simulink model "sampleModel106"  (R2022a)
settings: Solver=VariableStepAuto  StartTime=0.0  StopTime=10.0  RelTol=1e-3
undefined symbols (not defined in the file): DiscIntNeverNeededParam, magnitude, Newton, Raphson
libraries: simulink x379, slpidlib x89
(part 4 of 16)

== system sampleModel106/cfblk79/cfblk7/cfblk10 ==
  cfblk1 : Inport
  cfblk10 : Constant  Value=[930798698.879540]  SampleTime=1
  cfblk11 : Constant  Value=[942896576.125749]  SampleTime=1
  cfblk12 : Subsystem
  cfblk13 : Subsystem
  cfblk14 : Subsystem
  cfblk{15..18} (4 alike) : Delay  SampleTime=1
  cfblk3 : slpidlib/PID Controller (2DOF)  Controller=PID  Form=Parallel  TimeDomain=Discrete-time  UseExternalTs=off  SampleTime=1  IntegratorMethod=Forward Euler  FilterMethod=Forward Euler  ControllerParametersSource=internal  P=1  I=1  UseKiTs=off  D=0  N=100  UseFilter=on  b=1  c=1  TunerSelectOption=Transfer Function Based (PID Tuner App)  InitialConditionSource=internal  InitialConditionForIntegrator=0  InitialConditionForFilter=0  DifferentiatorICPrevScaledInput=0  ExternalReset=none  TrackingMode=off  Kt=1  LimitOutput=off  SatLimitsSource=internal  UpperSaturationLimit=inf  LowerSaturationLimit=-inf  LinearizeAsGain=off  AntiWindupMode=none  Kb=1  POutMin=[]  POutMax=[]  IOutMin=[]  IOutMax=[]  DOutMin=[]  DOutMax=[]  NOutMin=[]  NOutMax=[]  bOutMin=[]  bOutMax=[]  cOutMin=[]  cOutMax=[]  SumOutMin=[]  SumOutMax=[]  SaturationOutMin=[]  SaturationOutMax=[]  PParamMin=[]  PParamMax=[]  IParamMin=[]  IParamMax=[]  DParamMin=[]  DParamMax=[]  NParamMin=[]  NParamMax=[]  bParamMin=[]  bParamMax=[]  cParamMin=[]  cParamMax=[]  KbParamMin=[]  KbParamMax=[]  KtParamMin=[]  KtParamMax=[]  KbOutMin=[]  KbOutMax=[]  KtOutMin=[]  KtOutMax=[]  IntegratorOutMin=[]  IntegratorOutMax=[]  FilterOutMin=[]  FilterOutMax=[]  SumI1OutMin=[]  SumI1OutMax=[]  SumI2OutMin=[]  SumI2OutMax=[]  SumI3OutMin=[]  SumI3OutMax=[]  SumI4OutMin=[]  SumI4OutMax=[]  SumDOutMin=[]  SumDOutMax=[]  Sum1OutMin=[]  Sum1OutMax=[]  Sum2OutMin=[]  Sum2OutMax=[]  Sum3OutMin=[]  Sum3OutMax=[]  DifferentiatorOutMin=[]  DifferentiatorOutMax=[]  FilterDiffOutCoefMin=[]  FilterDiffOutCoefMax=[]  ReciprocalOutMin=[]  ReciprocalOutMax=[]  SumDenOutMin=[]  SumDenOutMax=[]  SumNumOutMin=[]  SumNumOutMax=[]  DivideOutMin=[]  DivideOutMax=[]  UdiffTsProdOutMin=[]  UdiffTsProdOutMax=[]  NTsProdOutMin=[]  NTsProdOutMax=[]  UintegralTsProdOutMin=[]  UintegralTsProdOutMax=[]  UngainTsProdOutMin=[]  UngainTsProdOutMax=[]  IntegratorContinuousStateAttributes=''  IntegratorStateMustResolveToSignalObject=off  IntegratorRTWStateStorageClass=Auto  FilterContinuousStateAttributes=''  FilterStateMustResolveToSignalObject=off  FilterRTWStateStorageClass=Auto  ParallelPVariant=InternalParameters  IdealPVariant=Disabled  IVariant=InternalParameters  DVariant=InternalParameters  bVariant=InternalParameters  cVariant=InternalParameters  IntegratorVariant=Discrete  SatVariant=Disabled  AWVariant=Passthrough  PCopyVariant=Disabled  TRVariant=Disabled  FdbkBlocksVariant=Forward  IdealPFdbkVariant=Disabled  SatFdbkVariant=Disabled  DerivativeFilterVariant=ForwardEulerFilter  NVariant=InternalParameters  NCopyVariant=Disabled  FilterICVariant=InternalICsFilter  IntegratorICVariant=InternalICs  ExternalResetVariant=Disabled  TRSumVariant=Passthrough  SumFdbkVariant=Disabled  SumVariant=Sum_PID  TsampFilterVariant=InternalTs  TsampNgainVariant=Passthrough  TsampIntegralVariant=Passthrough  ExternalSaturationOutDataTypeStr=Inherit: Same as second input
      settings: SourceProductBaseCode=SL
  cfblk4 : simulink/Discrete/Transfer Fcn Real Zero  ZeroZ=0.75  ICPrevInput=0.0  DoSatur=off
      settings: SourceProductBaseCode=SL
  cfblk5 : simulink/Discrete/Transfer Fcn First Order  PoleZ=0.95  ICPrevOutput=0.0  DoSatur=off
  cfblk6 : Sqrt
  cfblk7 : Sqrt
  cfblk8 : simulink/Math Operations/Slider Gain  gain=1  low=0  high=2
  cfblk9 : Bias  Bias=[-914547020.820806]  SaturateOnIntegerOverflow=off
  cfblk2 : Outport
  wires:
  cfblk5/1 -> cfblk9/1, cfblk12/2(cfblk9)
  cfblk7/1 -> cfblk4/1
  cfblk12/1(cfblk2) -> cfblk13/1(cfblk1)
  cfblk1/1 -> cfblk14/1(cfblk1)
  cfblk14/1(cfblk2) -> cfblk7/1
  cfblk13/1(cfblk2) -> cfblk3/1
  cfblk8/1 -> cfblk13/2(cfblk16)
  cfblk10/1 -> cfblk8/1
  cfblk9/1 -> cfblk6/1, cfblk18/1
  cfblk11/1 -> cfblk13/3(cfblk17)
  cfblk14/2(cfblk16) -> cfblk5/1
  cfblk14/3(cfblk17) -> cfblk3/2
  cfblk12/2(cfblk11) -> cfblk2/1
  cfblk4/1 -> cfblk12/1(cfblk1), cfblk12/3(cfblk10)
  cfblk3/1 -> cfblk15/1
  cfblk15/1 -> cfblk14/2(cfblk12)
  cfblk12/3(cfblk12) -> cfblk16/1
  cfblk16/1 -> cfblk14/4(cfblk14)
  cfblk6/1 -> cfblk17/1
  cfblk17/1 -> cfblk14/3(cfblk13)
  cfblk18/1 -> cfblk14/5(cfblk15)

== system sampleModel106/cfblk79/cfblk7/cfblk11 ==
  cfblk1 : Inport
  cfblk13 : Inport  Port=2
  cfblk14 : Inport  Port=3
  cfblk10 : Subsystem
  cfblk11 : Subsystem
  cfblk12 : Subsystem
  cfblk18 : Delay  SampleTime=1
  cfblk3 : simulink/Discrete/Transfer Fcn First Order  PoleZ=0.95  ICPrevOutput=0.0  DoSatur=off
  cfblk4 : Sqrt
  cfblk5 : Constant  Value=[-218946941.041430]  SampleTime=1
  cfblk6 : Constant  Value=[703044914.610683]  SampleTime=1
  cfblk7 : Constant  Value=[340158216.869012]  SampleTime=1
  cfblk8 : Constant  Value=[55648413.249553]  SampleTime=1
  cfblk9 : Subsystem
  cfblk2 : Outport
  cfblk15 : Outport  Port=2
  cfblk16 : Outport  Port=3
  cfblk17 : Outport  Port=4
  wires:
  cfblk9/1(cfblk2) -> cfblk12/1(cfblk1)
  cfblk1/1 -> cfblk3/1
  cfblk7/1 -> cfblk16/1
  cfblk9/2(cfblk13) -> cfblk11/1(cfblk1)
  cfblk9/3(cfblk14) -> cfblk4/1
  cfblk5/1 -> cfblk17/1, cfblk9/3(cfblk12)
  cfblk14/1 -> cfblk11/2(cfblk11)
  cfblk11/1(cfblk2) -> cfblk15/1
  cfblk11/2(cfblk13) -> cfblk10/1(cfblk1)
  cfblk6/1 -> cfblk2/1
  cfblk4/1 -> cfblk11/3(cfblk12), cfblk12/3(cfblk14)
  cfblk13/1 -> cfblk10/2(cfblk12)
  cfblk12/1(cfblk2) -> cfblk10/3(cfblk13)
  cfblk3/1 -> cfblk9/1(cfblk1)
  cfblk8/1 -> cfblk9/2(cfblk11)
  cfblk10/1(cfblk2) -> cfblk18/1
  cfblk18/1 -> cfblk12/2(cfblk13)

== system sampleModel106/cfblk79/cfblk7/cfblk12 ==
  cfblk1 : Inport
  cfblk15 : Inport  Port=2
  cfblk16 : Inport  Port=3
  cfblk10 : Constant  Value=[896827998.321361]  SampleTime=1
  cfblk11 : Subsystem
  cfblk12 : Subsystem
  cfblk13 : Subsystem
  cfblk14 : Subsystem
  cfblk{18..22} (5 alike) : Delay  SampleTime=1
  cfblk3 : ComplexToMagnitudeAngle
  cfblk4 : Product
  cfblk5 : Gain  Gain=[-931939284.867982]
  cfblk6 : simulink/Math Operations/MinMax Running Resettable  Function=min  vinit=0.0
  cfblk7 : Bias  Bias=[-319907071.485030]  SaturateOnIntegerOverflow=off
  cfblk8 : Sum  Inputs=+-
  cfblk9 : Constant  Value=[-736006589.998858]  SampleTime=1
  cfblk2 : Outport
  cfblk17 : Outport  Port=2
  wires:
  cfblk6/1 -> cfblk11/1(cfblk1)
  cfblk15/1 -> cfblk11/2(cfblk9)
  cfblk5/1 -> cfblk2/1
  cfblk1/1 -> cfblk3/1
  cfblk16/1 -> cfblk5/1
  cfblk3/1 -> cfblk17/1
  cfblk9/1 -> cfblk14/1(cfblk1)
  cfblk14/1(cfblk2) -> cfblk13/1(cfblk1)
  cfblk8/1 -> cfblk4/1
  cfblk3/2 -> cfblk8/2
  cfblk14/2(cfblk14) -> cfblk12/1(cfblk1)
  cfblk13/2(cfblk11) -> cfblk4/2
  cfblk13/3(cfblk12) -> cfblk7/1
  cfblk11/1(cfblk2) -> cfblk14/2(cfblk12)
  cfblk4/1 -> cfblk18/1
  cfblk18/1 -> cfblk8/1
  cfblk13/1(cfblk2) -> cfblk19/1
  cfblk19/1 -> cfblk6/1
  cfblk7/1 -> cfblk20/1
  cfblk20/1 -> cfblk13/2(cfblk10)
  cfblk12/1(cfblk2) -> cfblk21/1
  cfblk21/1 -> cfblk14/3(cfblk13)
  cfblk14/3(cfblk15) -> cfblk22/1
  cfblk22/1 -> cfblk6/2

== system sampleModel106/cfblk79/cfblk7/cfblk13 ==
  cfblk1 : Inport
  cfblk10 : Subsystem  TreatAsAtomicUnit=on
  cfblk{11..14} (4 alike) : Delay  SampleTime=1
  cfblk3 : MinMax  Inputs=2
  cfblk4 : PermuteDimensions
  cfblk5 : Constant  Value=[199750980.008427]  SampleTime=1
  cfblk6 : Subsystem
  cfblk7 : Subsystem
  cfblk8 : If  IfExpression=u1 >= 0  SampleTime=1
  cfblk9 : Subsystem  TreatAsAtomicUnit=on
  cfblk2 : Outport
  wires:
  cfblk3/1 -> cfblk10/1(cfblk1)
  cfblk10/1(cfblk2) -> cfblk2/1
  cfblk4/1 -> cfblk9/2(cfblk13)
  cfblk5/1 -> cfblk6/1(cfblk1)
  cfblk1/1 -> cfblk10/2(cfblk8)
  cfblk9/2(cfblk14) -> cfblk7/1(cfblk1)
  cfblk9/3(cfblk15) -> cfblk7/2(cfblk11)
  cfblk7/2(cfblk12) -> cfblk3/1
  cfblk6/2(cfblk7) -> cfblk3/2
  cfblk7/3(cfblk13) -> cfblk6/2(cfblk6)
  cfblk8/1 -> cfblk9/Action
  cfblk8/2 -> cfblk10/Action
  cfblk9/1(cfblk2) -> cfblk11/1
  cfblk11/1 -> cfblk4/1
  cfblk7/1(cfblk2) -> cfblk12/1
  cfblk12/1 -> cfblk9/1(cfblk1)
  cfblk6/1(cfblk2) -> cfblk13/1
  cfblk13/1 -> cfblk8/1
  cfblk7/4(cfblk14) -> cfblk14/1
  cfblk14/1 -> cfblk10/3(cfblk9)

== system sampleModel106/cfblk79/cfblk8/cfblk10 ==
  cfblk1 : Inport
  cfblk{3,11..17} (8 alike) : Delay  SampleTime=1
  cfblk4 : Delay  ShowEnablePort=on  SampleTime=1
      settings: InputPortMap=u0,e6
  cfblk5 : Abs  SaturateOnIntegerOverflow=off
  cfblk6 : Sqrt  Operator=rSqrt  AlgorithmType=Newton-Raphson
  cfblk7 : Subsystem
  cfblk8 : Subsystem
  cfblk2 : Outport
  cfblk9 : Outport  Port=2
  cfblk10 : Outport  Port=3
  wires:
  cfblk3/1 -> cfblk9/1
  cfblk6/1 -> cfblk5/1, cfblk2/1, cfblk16/1, cfblk17/1
  cfblk5/1 -> cfblk4/1, cfblk4/2, cfblk11/1, cfblk12/1
  cfblk1/1 -> cfblk7/2(cfblk6), cfblk8/3(cfblk10)
  cfblk7/1(cfblk2) -> cfblk8/1(cfblk1)
  cfblk8/1(cfblk2) -> cfblk10/1
  cfblk8/2(cfblk13) -> cfblk6/1
  cfblk8/3(cfblk14) -> cfblk3/1
  cfblk4/1 -> cfblk13/1, cfblk14/1, cfblk15/1
  cfblk11/1 -> cfblk7/1(cfblk1)
  cfblk12/1 -> cfblk7/3(cfblk7)
  cfblk13/1 -> cfblk8/2(cfblk9)
  cfblk14/1 -> cfblk8/4(cfblk11)
  cfblk15/1 -> cfblk7/5(cfblk9)
  cfblk16/1 -> cfblk8/5(cfblk12)
  cfblk17/1 -> cfblk7/4(cfblk8)

== system sampleModel106/cfblk79/cfblk8/cfblk11 ==
  cfblk1 : Inport
  cfblk14 : Inport  Port=2
  cfblk10 : Constant  Value=[476735084.227902]  SampleTime=1
  cfblk11 : Subsystem
  cfblk12 : Subsystem
  cfblk13 : If  IfExpression=u1 >= 0  SampleTime=1
  cfblk18 : Subsystem  TreatAsAtomicUnit=on
  cfblk19 : Subsystem  TreatAsAtomicUnit=on
  cfblk20 : Delay  SampleTime=1
  cfblk21 : Delay  SampleTime=1
  cfblk22 : Delay  SampleTime=1
  cfblk3 : simulink/Discrete/Transfer Fcn Real Zero  ZeroZ=0.75  ICPrevInput=0.0  DoSatur=off
      settings: SourceProductBaseCode=SL
  cfblk4 : Product  Inputs=**
  cfblk5 : Sqrt  Operator=rSqrt  AlgorithmType=Newton-Raphson
  cfblk6 : Signum
  cfblk7 : Signum
  cfblk8 : Sum  Inputs=+
  cfblk9 : Constant  Value=[-437500950.255498]  SampleTime=1
  cfblk2 : Outport
  cfblk15 : Outport  Port=2
  cfblk16 : Outport  Port=3
  cfblk17 : Outport  Port=4
  wires:
  cfblk8/1 -> cfblk11/1(cfblk1)
  cfblk3/1 -> cfblk5/1, cfblk11/3(cfblk13)
  cfblk7/1 -> cfblk15/1, cfblk21/1
  cfblk19/1(cfblk2) -> cfblk4/1
  cfblk19/2(cfblk13) -> cfblk16/1
  cfblk6/1 -> cfblk13/1
  cfblk12/1(cfblk2) -> cfblk7/1
  cfblk12/2(cfblk10) -> cfblk2/1
  cfblk19/3(cfblk14) -> cfblk17/1
  cfblk11/1(cfblk2) -> cfblk4/2
  cfblk10/1 -> cfblk8/1, cfblk19/3(cfblk12)
  cfblk19/4(cfblk15) -> cfblk3/1, cfblk11/4(cfblk14)
  cfblk5/1 -> cfblk12/1(cfblk1), cfblk11/6(cfblk16)
  cfblk18/1(cfblk2) -> cfblk11/2(cfblk12)
  cfblk14/1 -> cfblk12/2(cfblk9)
  cfblk1/1 -> cfblk6/1, cfblk11/5(cfblk15)
  cfblk9/1 -> cfblk19/2(cfblk11)
  cfblk13/1 -> cfblk18/Action
  cfblk13/2 -> cfblk19/Action
  cfblk4/1 -> cfblk20/1
  cfblk20/1 -> cfblk18/2(cfblk8)
  cfblk21/1 -> cfblk18/1(cfblk1)
  cfblk12/3(cfblk11) -> cfblk22/1
  cfblk22/1 -> cfblk19/1(cfblk1)

== system sampleModel106/cfblk79/cfblk8/cfblk9 ==
  cfblk1 : Inport
  cfblk10 : Inport  Port=2
  cfblk11 : Inport  Port=3
  cfblk12 : Inport  Port=4
  cfblk13 : Delay  SampleTime=1
  cfblk14 : Delay  SampleTime=1
  cfblk3 : simulink/Math Operations/MinMax Running Resettable  Function=min  vinit=0.0
  cfblk4 : Sqrt  Operator=rSqrt  AlgorithmType=Newton-Raphson
  cfblk5 : Signum
  cfblk6 : Polyval  Coefs=[ +2.081618890e-019, -1.441693666e-014, +4.719686976e-010, -8.536869453e-006, +1.621573104e-001, -8.087801117e+001 ]
  cfblk7 : Abs  SaturateOnIntegerOverflow=off
  cfblk8 : Sum  Inputs=--
  cfblk9 : Subsystem
  cfblk2 : Outport
  wires:
  cfblk11/1 -> cfblk2/1
  cfblk10/1 -> cfblk3/1
  cfblk4/1 -> cfblk6/1
  cfblk12/1 -> cfblk9/1(cfblk1)
  cfblk9/1(cfblk2) -> cfblk4/1
  cfblk8/1 -> cfblk3/2
  cfblk7/1 -> cfblk8/1
  cfblk6/1 -> cfblk8/2, cfblk14/1
  cfblk9/2(cfblk10) -> cfblk7/1
  cfblk1/1 -> cfblk5/1
  cfblk5/1 -> cfblk9/2(cfblk7)
  cfblk3/1 -> cfblk13/1
  cfblk13/1 -> cfblk9/3(cfblk8)
  cfblk14/1 -> cfblk9/4(cfblk9)

== system sampleModel106/cfblk80/cfblk10/cfblk10 ==
  cfblk1 : Inport
  cfblk13 : Inport  Port=2
  cfblk10 : Subsystem
  cfblk11 : Subsystem
  cfblk12 : Subsystem
  cfblk15 : Delay  SampleTime=1
  cfblk16 : Delay  SampleTime=1
  cfblk17 : Delay  SampleTime=1
  cfblk3 : ComplexToRealImag
  cfblk4 : Product  Inputs=*
  cfblk5 : simulink/Math Operations/Slider Gain  gain=1  low=0  high=2
  cfblk6 : PermuteDimensions
  cfblk7 : Trigonometry
  cfblk8 : Constant  Value=[898456945.035176]  SampleTime=1
  cfblk9 : Subsystem
  cfblk2 : Outport
  cfblk14 : Outport  Port=2
  wires:
  cfblk1/1 -> cfblk9/1(cfblk1)
  cfblk13/1 -> cfblk5/1
  cfblk10/1(cfblk2) -> cfblk12/1(cfblk1)
  cfblk10/2(cfblk7) -> cfblk7/1
  cfblk12/1(cfblk2) -> cfblk4/1
  cfblk8/1 -> cfblk11/1(cfblk1)
  cfblk9/1(cfblk2) -> cfblk6/1
  cfblk11/1(cfblk2) -> cfblk12/2(cfblk6), cfblk14/1
  cfblk6/1 -> cfblk10/1(cfblk1)
  cfblk5/1 -> cfblk2/1, cfblk3/1
  cfblk3/1 -> cfblk12/3(cfblk7)
  cfblk3/2 -> cfblk12/4(cfblk8), cfblk11/2(cfblk9)
  cfblk4/1 -> cfblk15/1
  cfblk15/1 -> cfblk9/3(cfblk13)
  cfblk12/2(cfblk9) -> cfblk16/1
  cfblk16/1 -> cfblk10/2(cfblk6)
  cfblk7/1 -> cfblk17/1
  cfblk17/1 -> cfblk9/2(cfblk12)

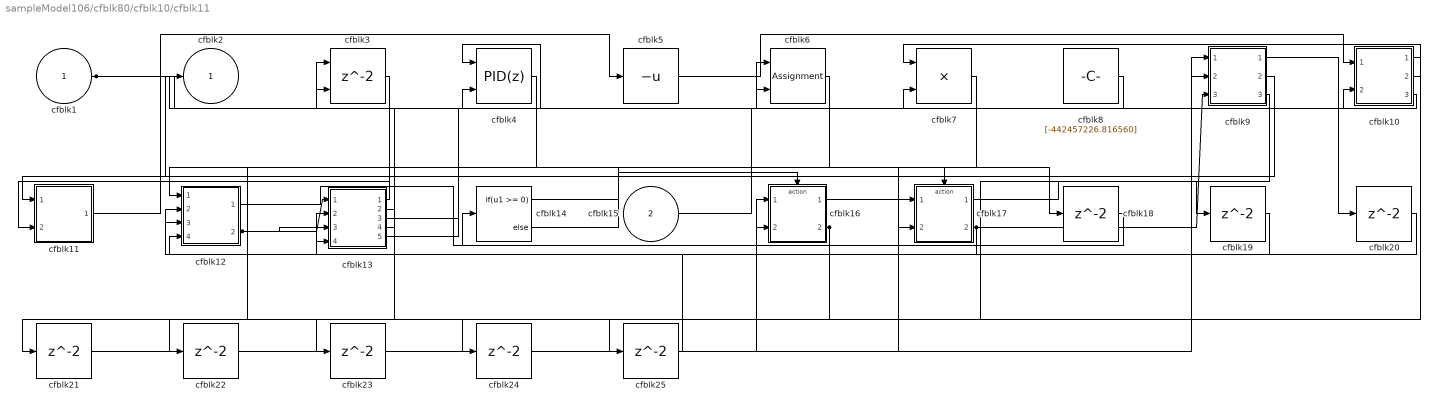
== system sampleModel106/cfblk80/cfblk10/cfblk11 ==
  cfblk1 : Inport
  cfblk15 : Inport  Port=2
  cfblk10 : Subsystem
  cfblk11 : Subsystem
  cfblk12 : Subsystem
  cfblk13 : Subsystem
  cfblk14 : If  IfExpression=u1 >= 0  SampleTime=1
  cfblk16 : Subsystem  TreatAsAtomicUnit=on
  cfblk17 : Subsystem  TreatAsAtomicUnit=on
  cfblk{18..25} (8 alike) : Delay  SampleTime=1
  cfblk3 : Delay  ShowEnablePort=on  SampleTime=1
      settings: InputPortMap=u0,e6
  cfblk4 : slpidlib/PID Controller (2DOF)  Controller=PID  Form=Parallel  TimeDomain=Discrete-time  UseExternalTs=off  SampleTime=1  IntegratorMethod=Forward Euler  FilterMethod=Forward Euler  ControllerParametersSource=internal  P=1  I=1  UseKiTs=off  D=0  N=100  UseFilter=on  b=1  c=1  TunerSelectOption=Transfer Function Based (PID Tuner App)  InitialConditionSource=internal  InitialConditionForIntegrator=0  InitialConditionForFilter=0  DifferentiatorICPrevScaledInput=0  ExternalReset=none  TrackingMode=off  Kt=1  LimitOutput=off  SatLimitsSource=internal  UpperSaturationLimit=inf  LowerSaturationLimit=-inf  LinearizeAsGain=off  AntiWindupMode=none  Kb=1  POutMin=[]  POutMax=[]  IOutMin=[]  IOutMax=[]  DOutMin=[]  DOutMax=[]  NOutMin=[]  NOutMax=[]  bOutMin=[]  bOutMax=[]  cOutMin=[]  cOutMax=[]  SumOutMin=[]  SumOutMax=[]  SaturationOutMin=[]  SaturationOutMax=[]  PParamMin=[]  PParamMax=[]  IParamMin=[]  IParamMax=[]  DParamMin=[]  DParamMax=[]  NParamMin=[]  NParamMax=[]  bParamMin=[]  bParamMax=[]  cParamMin=[]  cParamMax=[]  KbParamMin=[]  KbParamMax=[]  KtParamMin=[]  KtParamMax=[]  KbOutMin=[]  KbOutMax=[]  KtOutMin=[]  KtOutMax=[]  IntegratorOutMin=[]  IntegratorOutMax=[]  FilterOutMin=[]  FilterOutMax=[]  SumI1OutMin=[]  SumI1OutMax=[]  SumI2OutMin=[]  SumI2OutMax=[]  SumI3OutMin=[]  SumI3OutMax=[]  SumI4OutMin=[]  SumI4OutMax=[]  SumDOutMin=[]  SumDOutMax=[]  Sum1OutMin=[]  Sum1OutMax=[]  Sum2OutMin=[]  Sum2OutMax=[]  Sum3OutMin=[]  Sum3OutMax=[]  DifferentiatorOutMin=[]  DifferentiatorOutMax=[]  FilterDiffOutCoefMin=[]  FilterDiffOutCoefMax=[]  ReciprocalOutMin=[]  ReciprocalOutMax=[]  SumDenOutMin=[]  SumDenOutMax=[]  SumNumOutMin=[]  SumNumOutMax=[]  DivideOutMin=[]  DivideOutMax=[]  UdiffTsProdOutMin=[]  UdiffTsProdOutMax=[]  NTsProdOutMin=[]  NTsProdOutMax=[]  UintegralTsProdOutMin=[]  UintegralTsProdOutMax=[]  UngainTsProdOutMin=[]  UngainTsProdOutMax=[]  IntegratorContinuousStateAttributes=''  IntegratorStateMustResolveToSignalObject=off  IntegratorRTWStateStorageClass=Auto  FilterContinuousStateAttributes=''  FilterStateMustResolveToSignalObject=off  FilterRTWStateStorageClass=Auto  ParallelPVariant=InternalParameters  IdealPVariant=Disabled  IVariant=InternalParameters  DVariant=InternalParameters  bVariant=InternalParameters  cVariant=InternalParameters  IntegratorVariant=Discrete  SatVariant=Disabled  AWVariant=Passthrough  PCopyVariant=Disabled  TRVariant=Disabled  FdbkBlocksVariant=Forward  IdealPFdbkVariant=Disabled  SatFdbkVariant=Disabled  DerivativeFilterVariant=ForwardEulerFilter  NVariant=InternalParameters  NCopyVariant=Disabled  FilterICVariant=InternalICsFilter  IntegratorICVariant=InternalICs  ExternalResetVariant=Disabled  TRSumVariant=Passthrough  SumFdbkVariant=Disabled  SumVariant=Sum_PID  TsampFilterVariant=InternalTs  TsampNgainVariant=Passthrough  TsampIntegralVariant=Passthrough  ExternalSaturationOutDataTypeStr=Inherit: Same as second input
      settings: SourceProductBaseCode=SL
  cfblk5 : UnaryMinus
  cfblk6 : Assignment  DiagnosticForDimensions=Warning  IndexOptions=Index vector (dialog)  Indices=1  OutputSizes=1
  cfblk7 : Product  Inputs=**
  cfblk8 : Constant  Value=[-442457226.816560]  SampleTime=1
  cfblk9 : Subsystem
  cfblk2 : Outport
  wires:
  cfblk4/1 -> cfblk12/1(cfblk1)
  cfblk8/1 -> cfblk4/1
  cfblk11/1(cfblk2) -> cfblk5/1
  cfblk16/2(cfblk14) -> cfblk13/2(cfblk6), cfblk25/1
  cfblk5/1 -> cfblk10/1(cfblk1)
  cfblk1/1 -> cfblk4/2, cfblk17/2(cfblk11)
  cfblk12/1(cfblk2) -> cfblk16/1(cfblk1)
  cfblk10/2(cfblk11) -> cfblk7/1
  cfblk13/1(cfblk2) -> cfblk2/1
  cfblk9/2(cfblk9) -> cfblk11/1(cfblk1)
  cfblk15/1 -> cfblk10/2(cfblk10)
  cfblk17/2(cfblk12) -> cfblk9/3(cfblk8), cfblk13/4(cfblk8)
  cfblk13/2(cfblk9) -> cfblk3/1
  cfblk10/3(cfblk12) -> cfblk6/1
  cfblk13/3(cfblk10) -> cfblk6/2
  cfblk13/4(cfblk11) -> cfblk3/2
  cfblk13/5(cfblk12) -> cfblk7/2
  cfblk12/2(cfblk13) -> cfblk13/1(cfblk1), cfblk13/3(cfblk7)
  cfblk3/1 -> cfblk11/2(cfblk9)
  cfblk14/1 -> cfblk16/Action
  cfblk14/2 -> cfblk17/Action
  cfblk16/1(cfblk2) -> cfblk18/1
  cfblk18/1 -> cfblk14/1
  cfblk17/1(cfblk2) -> cfblk19/1
  cfblk19/1 -> cfblk12/3(cfblk11)
  cfblk9/1(cfblk2) -> cfblk20/1
  cfblk20/1 -> cfblk12/4(cfblk12)
  cfblk10/1(cfblk2) -> cfblk21/1
  cfblk21/1 -> cfblk9/2(cfblk7)
  cfblk7/1 -> cfblk22/1
  cfblk22/1 -> cfblk9/1(cfblk1)
  cfblk6/1 -> cfblk23/1
  cfblk23/1 -> cfblk16/2(cfblk13)
  cfblk9/3(cfblk10) -> cfblk24/1
  cfblk24/1 -> cfblk17/1(cfblk1)
  cfblk25/1 -> cfblk12/2(cfblk10)

== system sampleModel106/cfblk80/cfblk10/cfblk12 ==
  cfblk1 : Inport
  cfblk3 : Delay  ShowEnablePort=on  SampleTime=1
      settings: InputPortMap=u0,e6
  cfblk4 : Delay  ShowEnablePort=on  SampleTime=1
      settings: InputPortMap=u0,e6
  cfblk5 : slpidlib/PID Controller  Controller=PID  Form=Parallel  TimeDomain=Discrete-time  UseExternalTs=off  SampleTime=1  IntegratorMethod=Forward Euler  FilterMethod=Forward Euler  ControllerParametersSource=internal  P=1  I=1  UseKiTs=off  D=0  N=100  UseFilter=on  TunerSelectOption=Transfer Function Based (PID Tuner App)  InitialConditionSource=internal  InitialConditionForIntegrator=0  InitialConditionForFilter=0  DifferentiatorICPrevScaledInput=0  ExternalReset=none  TrackingMode=off  Kt=1  LimitOutput=off  SatLimitsSource=internal  UpperSaturationLimit=inf  LowerSaturationLimit=-inf  LinearizeAsGain=off  AntiWindupMode=none  Kb=1  POutMin=[]  POutMax=[]  IOutMin=[]  IOutMax=[]  DOutMin=[]  DOutMax=[]  NOutMin=[]  NOutMax=[]  SumOutMin=[]  SumOutMax=[]  SaturationOutMin=[]  SaturationOutMax=[]  PParamMin=[]  PParamMax=[]  IParamMin=[]  IParamMax=[]  DParamMin=[]  DParamMax=[]  NParamMin=[]  NParamMax=[]  KbParamMin=[]  KbParamMax=[]  KtParamMin=[]  KtParamMax=[]  KbOutMin=[]  KbOutMax=[]  KtOutMin=[]  KtOutMax=[]  IntegratorOutMin=[]  IntegratorOutMax=[]  FilterOutMin=[]  FilterOutMax=[]  SumI1OutMin=[]  SumI1OutMax=[]  SumI2OutMin=[]  SumI2OutMax=[]  SumI3OutMin=[]  SumI3OutMax=[]  SumI4OutMin=[]  SumI4OutMax=[]  SumDOutMin=[]  SumDOutMax=[]  DifferentiatorOutMin=[]  DifferentiatorOutMax=[]  FilterDiffOutCoefMin=[]  FilterDiffOutCoefMax=[]  ReciprocalOutMin=[]  ReciprocalOutMax=[]  SumDenOutMin=[]  SumDenOutMax=[]  SumNumOutMin=[]  SumNumOutMax=[]  DivideOutMin=[]  DivideOutMax=[]  UdiffTsProdOutMin=[]  UdiffTsProdOutMax=[]  NTsProdOutMin=[]  NTsProdOutMax=[]  UintegralTsProdOutMin=[]  UintegralTsProdOutMax=[]  UngainTsProdOutMin=[]  UngainTsProdOutMax=[]  IntegratorContinuousStateAttributes=''  IntegratorStateMustResolveToSignalObject=off  IntegratorRTWStateStorageClass=Auto  FilterContinuousStateAttributes=''  FilterStateMustResolveToSignalObject=off  FilterRTWStateStorageClass=Auto  ParallelPVariant=InternalParameters  IdealPVariant=Disabled  IVariant=InternalParameters  DVariant=InternalParameters  IntegratorVariant=Discrete  SatVariant=Disabled  AWVariant=Passthrough  PCopyVariant=Disabled  TRVariant=Disabled  FdbkBlocksVariant=Forward  IdealPFdbkVariant=Disabled  SatFdbkVariant=Disabled  DerivativeFilterVariant=ForwardEulerFilter  NVariant=InternalParameters  NCopyVariant=Disabled  FilterICVariant=InternalICsFilter  IntegratorICVariant=InternalICs  ExternalResetVariant=Disabled  TRSumVariant=Passthrough  SumFdbkVariant=Disabled  SumVariant=Sum_PID  TsampFilterVariant=InternalTs  TsampNgainVariant=Passthrough  TsampIntegralVariant=Passthrough  ExternalSaturationOutDataTypeStr=Inherit: Same as second input  aMode=0
  cfblk6 : Assignment  DiagnosticForDimensions=Warning  IndexOptions=Index vector (dialog)  Indices=1  OutputSizes=1
  cfblk7 : Sum  Inputs=+-
  cfblk8 : Constant  Value=[-633710361.624369]  SampleTime=1
  cfblk9 : Subsystem
  cfblk2 : Outport
  cfblk10 : Outport  Port=2
  cfblk11 : Outport  Port=3
  wires:
  cfblk7/1 -> cfblk2/1
  cfblk9/1(cfblk2) -> cfblk3/1
  cfblk5/1 -> cfblk10/1
  cfblk4/1 -> cfblk3/2
  cfblk3/1 -> cfblk5/1
  cfblk1/1 -> cfblk7/1, cfblk6/2
  cfblk8/1 -> cfblk9/1(cfblk1), cfblk4/1, cfblk11/1
  cfblk9/2(cfblk11) -> cfblk6/1, cfblk4/2
  cfblk6/1 -> cfblk7/2

== system sampleModel106/cfblk80/cfblk10/cfblk16 ==
  cfblk1 : Inport
  cfblk7 : Inport  Port=2
  Action Port : ActionPort  ActionPortLabel=if(u1 >= 0)
  cfblk3 : PermuteDimensions
  cfblk4 : Polyval  Coefs=[ +2.081618890e-019, -1.441693666e-014, +4.719686976e-010, -8.536869453e-006, +1.621573104e-001, -8.087801117e+001 ]
  cfblk5 : Sum  Inputs=+-
  cfblk6 : Subsystem
  cfblk8 : Delay
  cfblk9 : Delay
  cfblk2 : Outport
  wires:
  cfblk4/1 -> cfblk5/1
  cfblk6/1(cfblk2) -> cfblk3/1
  cfblk1/1 -> cfblk6/1(cfblk1)
  cfblk6/2(cfblk11) -> cfblk4/1
  cfblk5/1 -> cfblk8/1, cfblk9/1
  cfblk3/1 -> cfblk2/1, cfblk5/2
  cfblk7/1 -> cfblk6/3(cfblk8), cfblk6/5(cfblk10)
  cfblk8/1 -> cfblk6/2(cfblk7)
  cfblk9/1 -> cfblk6/4(cfblk9)

== system sampleModel106/cfblk80/cfblk10/cfblk17 ==
  cfblk1 : Inport
  cfblk16 : Inport  Port=2
  Action Port : ActionPort  ActionPortLabel=else
  cfblk10 : Trigonometry
  cfblk11 : Product  Inputs=**
  cfblk12 : Constant  Value=[9296872.569103]  SampleTime=1
  cfblk13 : Subsystem
  cfblk14 : Subsystem
  cfblk15 : Subsystem
  cfblk18 : Delay
  cfblk19 : Delay
  cfblk20 : Delay
  cfblk3 : simulink/Discrete/Transfer Fcn Lead or Lag  PoleZ=0.95  ZeroZ=0.75  ICPrevOutput=0.0  ICPrevInput=0.0  DoSatur=off
      settings: SourceProductBaseCode=SL
  cfblk4 : simulink/Discrete/Transfer Fcn Lead or Lag  PoleZ=0.95  ZeroZ=0.75  ICPrevOutput=0.0  ICPrevInput=0.0  DoSatur=off
      settings: SourceProductBaseCode=SL
  cfblk5 : DiscreteZeroPole  Poles=[0 0.5]  Gain=1  SampleTime=-1
  cfblk6 : DiscreteTransferFcn
  cfblk7 : PermuteDimensions
  cfblk8 : Reshape
  cfblk9 : Sqrt  Operator=rSqrt  AlgorithmType=Newton-Raphson
  cfblk2 : Outport
  cfblk17 : Outport  Port=2
  wires:
  cfblk6/1 -> cfblk7/1, cfblk20/1
  cfblk16/1 -> cfblk13/1(cfblk1)
  cfblk13/1(cfblk2) -> cfblk10/1
  cfblk13/2(cfblk15) -> cfblk2/1, cfblk15/3(cfblk10), cfblk14/5(cfblk11)
  cfblk14/1(cfblk2) -> cfblk3/1
  cfblk7/1 -> cfblk4/1, cfblk19/1
  cfblk10/1 -> cfblk5/1
  cfblk12/1 -> cfblk14/1(cfblk1)
  cfblk11/1 -> cfblk13/2(cfblk14)
  cfblk1/1 -> cfblk11/1
  cfblk3/1 -> cfblk17/1
  cfblk5/1 -> cfblk14/2(cfblk8)
  cfblk15/1(cfblk2) -> cfblk6/1
  cfblk9/1 -> cfblk14/3(cfblk9), cfblk14/6(cfblk12)
  cfblk4/1 -> cfblk9/1, cfblk8/1
  cfblk8/1 -> cfblk14/4(cfblk10)
  cfblk14/2(cfblk13) -> cfblk18/1
  cfblk18/1 -> cfblk11/2
  cfblk19/1 -> cfblk15/2(cfblk9)
  cfblk20/1 -> cfblk15/1(cfblk1)

== system sampleModel106/cfblk80/cfblk10/cfblk7 ==
  cfblk1 : Inport
  cfblk10 : If  IfExpression=u1 >= 0  SampleTime=1
  cfblk11 : Subsystem  TreatAsAtomicUnit=on
  cfblk12 : Subsystem  TreatAsAtomicUnit=on
  cfblk{13..16} (4 alike) : Delay  SampleTime=1
  cfblk3 : simulink/Discrete/Tapped Delay  vinit=0.0  samptime=-1  NumDelays=1  DelayOrder=Oldest  includeCurrent=off
  cfblk4 : simulink/Math Operations/Slider Gain  gain=1  low=0  high=2
  cfblk5 : Sqrt
  cfblk6 : Product  Inputs=**
  cfblk7 : Subsystem
  cfblk8 : Subsystem
  cfblk9 : Subsystem
  cfblk2 : Outport
  wires:
  cfblk4/1 -> cfblk9/1(cfblk1)
  cfblk3/1 -> cfblk10/1
  cfblk7/1(cfblk2) -> cfblk8/1(cfblk1)
  cfblk11/2(cfblk12) -> cfblk12/1(cfblk1)
  cfblk1/1 -> cfblk7/1(cfblk1)
  cfblk12/1(cfblk2) -> cfblk5/1
  cfblk12/2(cfblk7) -> cfblk2/1
  cfblk9/2(cfblk12) -> cfblk6/1
  cfblk9/3(cfblk13) -> cfblk6/2
  cfblk7/2(cfblk12) -> cfblk8/2(cfblk10)
  cfblk6/1 -> cfblk8/3(cfblk11)
  cfblk10/1 -> cfblk11/Action
  cfblk10/2 -> cfblk12/Action
  cfblk8/1(cfblk2) -> cfblk13/1
  cfblk13/1 -> cfblk7/2(cfblk11)
  cfblk11/1(cfblk2) -> cfblk14/1
  cfblk14/1 -> cfblk3/1
  cfblk5/1 -> cfblk15/1
  cfblk15/1 -> cfblk11/1(cfblk1)
  cfblk9/1(cfblk2) -> cfblk16/1
  cfblk16/1 -> cfblk4/1

== system sampleModel106/cfblk80/cfblk10/cfblk8 ==
  cfblk1 : Inport
  cfblk10 : Subsystem
  cfblk11 : If  IfExpression=u1 >= 0  SampleTime=1
  cfblk12 : Subsystem  TreatAsAtomicUnit=on
  cfblk13 : Subsystem  TreatAsAtomicUnit=on
  cfblk{14..21} (8 alike) : Delay  SampleTime=1
  cfblk3 : simulink/Discrete/Transfer Fcn Real Zero  ZeroZ=0.75  ICPrevInput=0.0  DoSatur=off
      settings: SourceProductBaseCode=SL
  cfblk4 : Assignment  DiagnosticForDimensions=Warning  IndexOptions=Index vector (dialog)  Indices=1  OutputSizes=1
  cfblk5 : Constant  Value=[-476104574.584805]  SampleTime=1
  cfblk6 : Subsystem
  cfblk7 : Subsystem
  cfblk8 : Subsystem
  cfblk9 : Subsystem
  cfblk2 : Outport
  wires:
  cfblk4/1 -> cfblk8/4(cfblk9), cfblk20/1, cfblk21/1
  cfblk6/1(cfblk2) -> cfblk8/1(cfblk1)
  cfblk13/1(cfblk2) -> cfblk2/1
  cfblk1/1 -> cfblk10/1(cfblk1)
  cfblk10/1(cfblk2) -> cfblk12/1(cfblk1)
  cfblk10/2(cfblk8) -> cfblk3/1
  cfblk8/1(cfblk2) -> cfblk7/1(cfblk1)
  cfblk5/1 -> cfblk13/2(cfblk13)
  cfblk7/1(cfblk2) -> cfblk9/1(cfblk1)
  cfblk3/1 -> cfblk9/2(cfblk7), cfblk6/3(cfblk9), cfblk6/4(cfblk10), cfblk8/3(cfblk8)
  cfblk12/1(cfblk2) -> cfblk6/1(cfblk1)
  cfblk12/2(cfblk15) -> cfblk6/2(cfblk8)
  cfblk8/2(cfblk10) -> cfblk7/3(cfblk16)
  cfblk12/3(cfblk16) -> cfblk4/1
  cfblk12/4(cfblk17) -> cfblk4/2, cfblk13/6(cfblk17)
  cfblk8/4(cfblk12) -> cfblk18/1, cfblk19/1
  cfblk11/1 -> cfblk12/Action
  cfblk11/2 -> cfblk13/Action
  cfblk9/1(cfblk2) -> cfblk14/1
  cfblk14/1 -> cfblk8/2(cfblk7)
  cfblk9/2(cfblk8) -> cfblk15/1
  cfblk15/1 -> cfblk12/2(cfblk14)
  cfblk9/3(cfblk9) -> cfblk16/1
  cfblk16/1 -> cfblk7/2(cfblk15)
  cfblk8/3(cfblk11) -> cfblk17/1
  cfblk17/1 -> cfblk13/3(cfblk14)
  cfblk18/1 -> cfblk11/1
  cfblk19/1 -> cfblk13/5(cfblk16)
  cfblk20/1 -> cfblk13/1(cfblk1)
  cfblk21/1 -> cfblk13/4(cfblk15)

== system sampleModel106/cfblk80/cfblk10/cfblk9 ==
  cfblk1 : Inport
  cfblk10 : Inport  Port=2
  cfblk11 : Inport  Port=3
  cfblk12 : Delay  SampleTime=1
  cfblk3 : Sqrt  Operator=rSqrt  AlgorithmType=Newton-Raphson
  cfblk4 : ComplexToMagnitudeAngle
  cfblk5 : Product
  cfblk6 : Constant  Value=[774317516.290612]  SampleTime=1
  cfblk7 : Constant  Value=[275204604.701016]  SampleTime=1
  cfblk8 : Subsystem
  cfblk9 : Subsystem
  cfblk2 : Outport
  wires:
  cfblk5/1 -> cfblk4/1
  cfblk1/1 -> cfblk9/1(cfblk1)
  cfblk9/1(cfblk2) -> cfblk2/1
  cfblk7/1 -> cfblk3/1
  cfblk11/1 -> cfblk8/1(cfblk1)
  cfblk3/1 -> cfblk5/1
  cfblk4/1 -> cfblk8/2(cfblk7)
  cfblk10/1 -> cfblk8/3(cfblk8)
  cfblk6/1 -> cfblk8/4(cfblk9)
  cfblk8/1(cfblk2) -> cfblk12/1
  cfblk12/1 -> cfblk5/2

== system sampleModel106/cfblk80/cfblk11/cfblk10 ==
  cfblk1 : Inport
  cfblk10 : Delay  SampleTime=1
  cfblk11 : Delay  SampleTime=1
  cfblk3 : simulink/Discrete/Transfer Fcn Lead or Lag  PoleZ=0.95  ZeroZ=0.75  ICPrevOutput=0.0  ICPrevInput=0.0  DoSatur=off
      settings: SourceProductBaseCode=SL
  cfblk4 : Abs  SaturateOnIntegerOverflow=off
  cfblk5 : Gain  Gain=[471372579.211610]
  cfblk6 : ComplexToMagnitudeAngle
  cfblk7 : Sqrt  Operator=rSqrt  AlgorithmType=Newton-Raphson
  cfblk8 : Subsystem
  cfblk9 : Subsystem
  cfblk2 : Outport
  wires:
  cfblk9/1(cfblk2) -> cfblk5/1
  cfblk6/1 -> cfblk7/1
  cfblk3/1 -> cfblk6/1
  cfblk6/2 -> cfblk8/1(cfblk1)
  cfblk7/1 -> cfblk9/1(cfblk1)
  cfblk1/1 -> cfblk4/1
  cfblk4/1 -> cfblk2/1
  cfblk9/2(cfblk7) -> cfblk8/2(cfblk8)
  cfblk5/1 -> cfblk10/1
  cfblk10/1 -> cfblk3/1
  cfblk8/1(cfblk2) -> cfblk11/1
  cfblk11/1 -> cfblk9/2(cfblk6)

== system sampleModel106/cfblk80/cfblk11/cfblk8 ==
  cfblk1 : Inport
  cfblk13 : Inport  Port=2
  cfblk14 : Inport  Port=3
  cfblk15 : Inport  Port=4
  cfblk10 : Subsystem
  cfblk11 : Subsystem
  cfblk12 : Subsystem
  cfblk{16..20} (5 alike) : Delay  SampleTime=1
  cfblk3 : UnitDelay  HasFrameUpgradeWarning=on
  cfblk4 : Rounding
  cfblk5 : Product
  cfblk6 : Constant  Value=[721982136.145627]  SampleTime=1
  cfblk7 : Subsystem
  cfblk8 : Subsystem
  cfblk9 : Subsystem
  cfblk2 : Outport
  wires:
  cfblk12/1(cfblk2) -> cfblk10/1(cfblk1)
  cfblk15/1 -> cfblk9/1(cfblk1)
  cfblk11/1(cfblk2) -> cfblk9/2(cfblk11)
  cfblk3/1 -> cfblk5/1
  cfblk10/1(cfblk2) -> cfblk2/1
  cfblk6/1 -> cfblk11/1(cfblk1)
  cfblk13/1 -> cfblk5/2
  cfblk14/1 -> cfblk12/1(cfblk1)
  cfblk7/1(cfblk2) -> cfblk12/2(cfblk10), cfblk10/3(cfblk11)
  cfblk4/1 -> cfblk7/1(cfblk1)
  cfblk1/1 -> cfblk4/1
  cfblk11/2(cfblk11) -> cfblk8/1(cfblk1)
  cfblk10/2(cfblk12) -> cfblk8/4(cfblk15), cfblk16/1, cfblk17/1
  cfblk11/3(cfblk12) -> cfblk9/4(cfblk13), cfblk8/3(cfblk14)
  cfblk12/2(cfblk13) -> cfblk8/2(cfblk13)
  cfblk8/1(cfblk2) -> cfblk9/5(cfblk14)
  cfblk9/2(cfblk15) -> cfblk3/1, cfblk20/1
  cfblk16/1 -> cfblk7/2(cfblk7)
  cfblk17/1 -> cfblk12/3(cfblk11)
  cfblk9/1(cfblk2) -> cfblk18/1
  cfblk18/1 -> cfblk10/2(cfblk10)
  cfblk5/1 -> cfblk19/1
  cfblk19/1 -> cfblk9/3(cfblk12)
  cfblk20/1 -> cfblk12/4(cfblk12)

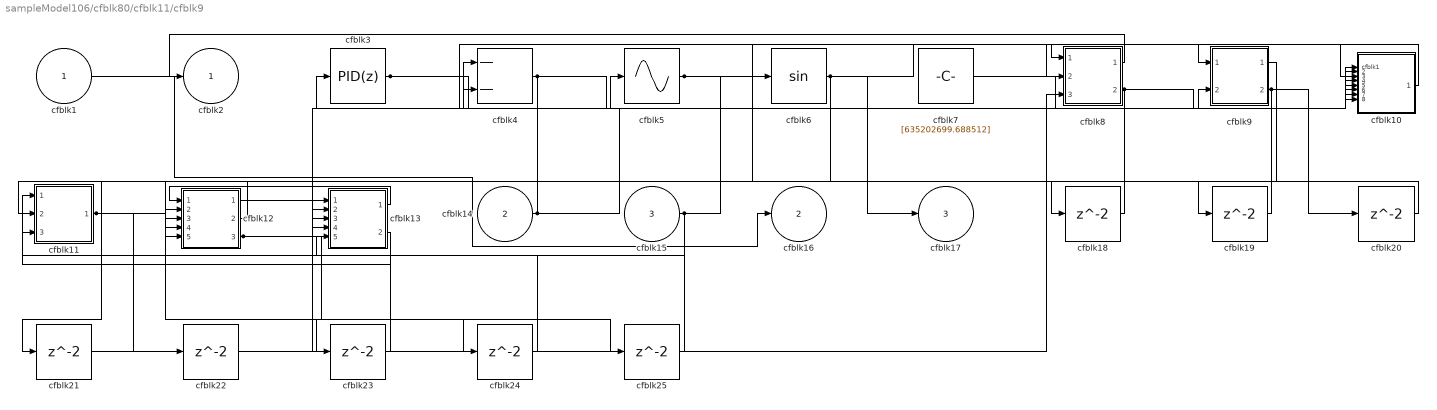
== system sampleModel106/cfblk80/cfblk11/cfblk9 ==
  cfblk1 : Inport
  cfblk14 : Inport  Port=2
  cfblk15 : Inport  Port=3
  cfblk10 : Subsystem
  cfblk11 : Subsystem
  cfblk12 : Subsystem
  cfblk13 : Subsystem
  cfblk{18..25} (8 alike) : Delay  SampleTime=1
  cfblk3 : slpidlib/PID Controller  Controller=PID  Form=Parallel  TimeDomain=Discrete-time  UseExternalTs=off  SampleTime=1  IntegratorMethod=Forward Euler  FilterMethod=Forward Euler  ControllerParametersSource=internal  P=1  I=1  UseKiTs=off  D=0  N=100  UseFilter=on  TunerSelectOption=Transfer Function Based (PID Tuner App)  InitialConditionSource=internal  InitialConditionForIntegrator=0  InitialConditionForFilter=0  DifferentiatorICPrevScaledInput=0  ExternalReset=none  TrackingMode=off  Kt=1  LimitOutput=off  SatLimitsSource=internal  UpperSaturationLimit=inf  LowerSaturationLimit=-inf  LinearizeAsGain=off  AntiWindupMode=none  Kb=1  POutMin=[]  POutMax=[]  IOutMin=[]  IOutMax=[]  DOutMin=[]  DOutMax=[]  NOutMin=[]  NOutMax=[]  SumOutMin=[]  SumOutMax=[]  SaturationOutMin=[]  SaturationOutMax=[]  PParamMin=[]  PParamMax=[]  IParamMin=[]  IParamMax=[]  DParamMin=[]  DParamMax=[]  NParamMin=[]  NParamMax=[]  KbParamMin=[]  KbParamMax=[]  KtParamMin=[]  KtParamMax=[]  KbOutMin=[]  KbOutMax=[]  KtOutMin=[]  KtOutMax=[]  IntegratorOutMin=[]  IntegratorOutMax=[]  FilterOutMin=[]  FilterOutMax=[]  SumI1OutMin=[]  SumI1OutMax=[]  SumI2OutMin=[]  SumI2OutMax=[]  SumI3OutMin=[]  SumI3OutMax=[]  SumI4OutMin=[]  SumI4OutMax=[]  SumDOutMin=[]  SumDOutMax=[]  DifferentiatorOutMin=[]  DifferentiatorOutMax=[]  FilterDiffOutCoefMin=[]  FilterDiffOutCoefMax=[]  ReciprocalOutMin=[]  ReciprocalOutMax=[]  SumDenOutMin=[]  SumDenOutMax=[]  SumNumOutMin=[]  SumNumOutMax=[]  DivideOutMin=[]  DivideOutMax=[]  UdiffTsProdOutMin=[]  UdiffTsProdOutMax=[]  NTsProdOutMin=[]  NTsProdOutMax=[]  UintegralTsProdOutMin=[]  UintegralTsProdOutMax=[]  UngainTsProdOutMin=[]  UngainTsProdOutMax=[]  IntegratorContinuousStateAttributes=''  IntegratorStateMustResolveToSignalObject=off  IntegratorRTWStateStorageClass=Auto  FilterContinuousStateAttributes=''  FilterStateMustResolveToSignalObject=off  FilterRTWStateStorageClass=Auto  ParallelPVariant=InternalParameters  IdealPVariant=Disabled  IVariant=InternalParameters  DVariant=InternalParameters  IntegratorVariant=Discrete  SatVariant=Disabled  AWVariant=Passthrough  PCopyVariant=Disabled  TRVariant=Disabled  FdbkBlocksVariant=Forward  IdealPFdbkVariant=Disabled  SatFdbkVariant=Disabled  DerivativeFilterVariant=ForwardEulerFilter  NVariant=InternalParameters  NCopyVariant=Disabled  FilterICVariant=InternalICsFilter  IntegratorICVariant=InternalICs  ExternalResetVariant=Disabled  TRSumVariant=Passthrough  SumFdbkVariant=Disabled  SumVariant=Sum_PID  TsampFilterVariant=InternalTs  TsampNgainVariant=Passthrough  TsampIntegralVariant=Passthrough  ExternalSaturationOutDataTypeStr=Inherit: Same as second input  aMode=0
  cfblk4 : Sum  Inputs=--
  cfblk5 : Sin  TimeSource=Use external signal  SampleTime=0
  cfblk6 : Trigonometry
  cfblk7 : Constant  Value=[635202699.688512]  SampleTime=1
  cfblk8 : Subsystem
  cfblk9 : Subsystem
  cfblk2 : Outport
  cfblk16 : Outport  Port=2
  cfblk17 : Outport  Port=3
  wires:
  cfblk5/1 -> cfblk8/1(cfblk1), cfblk18/1
  cfblk6/1 -> cfblk17/1, cfblk12/4(cfblk12), cfblk10/3(cfblk12), cfblk12/5(cfblk13)
  cfblk15/1 -> cfblk6/1, cfblk11/3(cfblk14)
  cfblk14/1 -> cfblk4/1, cfblk10/2(cfblk11)
  cfblk13/1(cfblk2) -> cfblk12/1(cfblk1)
  cfblk11/1(cfblk2) -> cfblk22/1, cfblk23/1
  cfblk1/1 -> cfblk16/1
  cfblk10/1(cfblk2) -> cfblk9/1(cfblk1)
  cfblk13/2(cfblk16) -> cfblk11/1(cfblk1)
  cfblk7/1 -> cfblk10/1(cfblk1)
  cfblk3/1 -> cfblk5/1, cfblk8/2(cfblk11), cfblk10/8(cfblk17)
  cfblk12/1(cfblk2) -> cfblk9/2(cfblk11)
  cfblk8/1(cfblk2) -> cfblk2/1
  cfblk4/1 -> cfblk13/3(cfblk13), cfblk10/5(cfblk14)
  cfblk8/2(cfblk13) -> cfblk4/2, cfblk10/4(cfblk13), cfblk10/6(cfblk15), cfblk10/7(cfblk16)
  cfblk9/2(cfblk12) -> cfblk20/1, cfblk21/1
  cfblk12/2(cfblk14) -> cfblk11/2(cfblk13)
  cfblk12/3(cfblk15) -> cfblk24/1, cfblk25/1
  cfblk18/1 -> cfblk3/1
  cfblk9/1(cfblk2) -> cfblk19/1
  cfblk19/1 -> cfblk13/2(cfblk12)
  cfblk20/1 -> cfblk12/2(cfblk10)
  cfblk21/1 -> cfblk8/3(cfblk12)
  cfblk22/1 -> cfblk13/1(cfblk1)
  cfblk23/1 -> cfblk12/3(cfblk11)
  cfblk24/1 -> cfblk13/4(cfblk14)
  cfblk25/1 -> cfblk13/5(cfblk15)

== system sampleModel106/cfblk80/cfblk12/cfblk9 ==
  cfblk1 : Inport
  cfblk{10..14} (5 alike) : Delay  SampleTime=1
  cfblk3 : Sum  Inputs=|++
  cfblk4 : Polyval  Coefs=[ +2.081618890e-019, -1.441693666e-014, +4.719686976e-010, -8.536869453e-006, +1.621573104e-001, -8.087801117e+001 ]
  cfblk5 : Constant  Value=[-791797657.618708]  SampleTime=1
  cfblk6 : Subsystem
  cfblk7 : If  IfExpression=u1 >= 0  SampleTime=1
  cfblk8 : Subsystem  TreatAsAtomicUnit=on
  cfblk9 : Subsystem  TreatAsAtomicUnit=on
  cfblk2 : Outport
  wires:
  cfblk6/1(cfblk2) -> cfblk12/1, cfblk13/1
  cfblk3/1 -> cfblk9/1(cfblk1)
  cfblk1/1 -> cfblk3/2
  cfblk5/1 -> cfblk9/2(cfblk9), cfblk9/5(cfblk12)
  cfblk8/3(cfblk14) -> cfblk6/1(cfblk1)
  cfblk9/1(cfblk2) -> cfblk4/1
  cfblk9/2(cfblk14) -> cfblk2/1
  cfblk9/3(cfblk15) -> cfblk8/1(cfblk1)
  cfblk9/4(cfblk16) -> cfblk8/2(cfblk12)
  cfblk7/1 -> cfblk8/Action
  cfblk7/2 -> cfblk9/Action
  cfblk8/1(cfblk2) -> cfblk10/1
  cfblk10/1 -> cfblk9/3(cfblk10)
  cfblk8/2(cfblk13) -> cfblk11/1
  cfblk11/1 -> cfblk9/4(cfblk11)
  cfblk12/1 -> cfblk3/1
  cfblk13/1 -> cfblk9/6(cfblk13)
  cfblk4/1 -> cfblk14/1
  cfblk14/1 -> cfblk7/1

== system sampleModel106/cfblk80/cfblk8/cfblk7 ==
  cfblk1 : Inport
  cfblk7 : Inport  Port=2
  cfblk3 : simulink/Discrete/Transfer Fcn First Order  PoleZ=0.95  ICPrevOutput=0.0  DoSatur=off
  cfblk4 : Math  Operator=10^u
  cfblk5 : Product
  cfblk6 : Subsystem
  cfblk8 : Delay  SampleTime=1
  cfblk9 : Delay  SampleTime=1
  cfblk2 : Outport
  wires:
  cfblk4/1 -> cfblk3/1
  cfblk3/1 -> cfblk5/1
  cfblk6/1(cfblk2) -> cfblk4/1
  cfblk6/2(cfblk12) -> cfblk2/1
  cfblk7/1 -> cfblk5/2, cfblk6/4(cfblk11)
  cfblk1/1 -> cfblk6/1(cfblk1)
  cfblk5/1 -> cfblk8/1, cfblk9/1
  cfblk8/1 -> cfblk6/2(cfblk9)
  cfblk9/1 -> cfblk6/3(cfblk10)

== system sampleModel106/cfblk80/cfblk8/cfblk8 ==
  cfblk1 : Inport
  cfblk10 : Delay  SampleTime=1
  cfblk3 : simulink/Discrete/Transfer Fcn Lead or Lag  PoleZ=0.95  ZeroZ=0.75  ICPrevOutput=0.0  ICPrevInput=0.0  DoSatur=off
      settings: SourceProductBaseCode=SL
  cfblk4 : UnitDelay  HasFrameUpgradeWarning=on
  cfblk5 : Constant  Value=[407730909.232018]  SampleTime=1
  cfblk6 : Subsystem
  cfblk7 : Subsystem
  cfblk8 : Delay  SampleTime=1
  cfblk9 : Delay  SampleTime=1
  cfblk2 : Outport
  wires:
  cfblk7/1(cfblk2) -> cfblk2/1
  cfblk1/1 -> cfblk3/1
  cfblk5/1 -> cfblk7/1(cfblk1), cfblk7/4(cfblk12), cfblk7/5(cfblk13)
  cfblk3/1 -> cfblk4/1, cfblk7/3(cfblk11)
  cfblk4/1 -> cfblk6/1(cfblk1), cfblk6/4(cfblk13)
  cfblk7/2(cfblk14) -> cfblk8/1, cfblk9/1, cfblk10/1
  cfblk6/1(cfblk2) -> cfblk7/2(cfblk10)
  cfblk8/1 -> cfblk6/2(cfblk11)
  cfblk9/1 -> cfblk6/3(cfblk12)
  cfblk10/1 -> cfblk6/5(cfblk14)

== system sampleModel106/cfblk80/cfblk9/cfblk11 ==
  cfblk1 : Inport
  cfblk10 : Inport  Port=2
  Action Port : ActionPort  ActionPortLabel=if(u1 >= 0)
  cfblk12 : Delay
  cfblk3 : Delay
  cfblk4 : simulink/Discrete/Transfer Fcn Real Zero  ZeroZ=0.75  ICPrevInput=0.0  DoSatur=off
      settings: SourceProductBaseCode=SL
  cfblk5 : simulink/Discrete/Transfer Fcn Lead or Lag  PoleZ=0.95  ZeroZ=0.75  ICPrevOutput=0.0  ICPrevInput=0.0  DoSatur=off
      settings: SourceProductBaseCode=SL
  cfblk6 : simulink/Discrete/Transfer Fcn Lead or Lag  PoleZ=0.95  ZeroZ=0.75  ICPrevOutput=0.0  ICPrevInput=0.0  DoSatur=off
      settings: SourceProductBaseCode=SL
  cfblk7 : Abs  SaturateOnIntegerOverflow=off
  cfblk8 : Abs  SaturateOnIntegerOverflow=off
  cfblk9 : Subsystem
  cfblk2 : Outport
  cfblk11 : Outport  Port=2
  wires:
  cfblk10/1 -> cfblk5/1
  cfblk5/1 -> cfblk4/1
  cfblk1/1 -> cfblk9/1(cfblk1)
  cfblk6/1 -> cfblk2/1
  cfblk3/1 -> cfblk6/1
  cfblk7/1 -> cfblk3/1, cfblk9/3(cfblk13)
  cfblk9/1(cfblk2) -> cfblk11/1
  cfblk4/1 -> cfblk7/1
  cfblk9/2(cfblk14) -> cfblk8/1
  cfblk8/1 -> cfblk12/1
  cfblk12/1 -> cfblk9/2(cfblk12)

== system sampleModel106/cfblk80/cfblk9/cfblk12 ==
  cfblk1 : Inport
  Action Port : ActionPort  ActionPortLabel=else
  cfblk10 : Subsystem
  cfblk11 : Subsystem
  cfblk{12..17} (6 alike) : Delay
  cfblk3 : simulink/Math Operations/Slider Gain  gain=1  low=0  high=2
  cfblk4 : simulink/Math Operations/MinMax Running Resettable  Function=min  vinit=0.0
  cfblk5 : Signum
  cfblk6 : Subsystem
  cfblk7 : Subsystem
  cfblk8 : Subsystem
  cfblk9 : Subsystem
  cfblk2 : Outport
  wires:
  cfblk10/1(cfblk2) -> cfblk6/1(cfblk1)
  cfblk4/1 -> cfblk9/1(cfblk1), cfblk11/2(cfblk8), cfblk15/1
  cfblk7/2(cfblk13) -> cfblk3/1, cfblk17/1
  cfblk6/1(cfblk2) -> cfblk8/1(cfblk1)
  cfblk6/2(cfblk10) -> cfblk7/1(cfblk1)
  cfblk10/2(cfblk12) -> cfblk4/1
  cfblk1/1 -> cfblk2/1, cfblk10/2(cfblk9)
  cfblk5/1 -> cfblk11/1(cfblk1)
  cfblk10/3(cfblk13) -> cfblk8/3(cfblk10)
  cfblk3/1 -> cfblk8/4(cfblk11), cfblk11/3(cfblk9), cfblk11/4(cfblk10)
  cfblk8/1(cfblk2) -> cfblk4/2
  cfblk8/2(cfblk14) -> cfblk5/1
  cfblk9/1(cfblk2) -> cfblk12/1
  cfblk12/1 -> cfblk8/2(cfblk9)
  cfblk11/1(cfblk2) -> cfblk13/1
  cfblk13/1 -> cfblk8/5(cfblk12)
  cfblk11/2(cfblk11) -> cfblk14/1
  cfblk14/1 -> cfblk8/6(cfblk13)
  cfblk15/1 -> cfblk10/4(cfblk11)
  cfblk7/1(cfblk2) -> cfblk16/1
  cfblk16/1 -> cfblk10/1(cfblk1)
  cfblk17/1 -> cfblk10/3(cfblk10)

== system sampleModel106/cfblk80/cfblk9/cfblk6 ==
  cfblk1 : Inport
  cfblk15 : Inport  Port=2
  cfblk16 : Inport  Port=3
  cfblk10 : Constant  Value=[-693339984.338294]  SampleTime=1
  cfblk11 : Subsystem
  cfblk12 : Subsystem
  cfblk13 : Subsystem
  cfblk14 : Subsystem
  cfblk17 : Delay  SampleTime=1
  cfblk3 : Delay  DelayLengthSource=Input port  SampleTime=1
      settings: InputPortMap=u0,p1
  cfblk4 : Sin  TimeSource=Use external signal  SampleTime=0
  cfblk5 : simulink/Math Operations/MinMax Running Resettable  Function=min  vinit=0.0
  cfblk6 : Abs  SaturateOnIntegerOverflow=off
  cfblk7 : Rounding
  cfblk8 : Reshape
  cfblk9 : Constant  Value=[-225892465.058717]  SampleTime=1
  cfblk2 : Outport
  wires:
  cfblk11/1(cfblk2) -> cfblk8/1
  cfblk4/1 -> cfblk13/1(cfblk1)
  cfblk13/1(cfblk2) -> cfblk7/1
  cfblk16/1 -> cfblk5/1, cfblk14/6(cfblk14)
  cfblk10/1 -> cfblk11/1(cfblk1)
  cfblk12/1(cfblk2) -> cfblk3/1
  cfblk15/1 -> cfblk13/3(cfblk9), cfblk14/4(cfblk12)
  cfblk9/1 -> cfblk11/2(cfblk12)
  cfblk11/2(cfblk13) -> cfblk3/2
  cfblk14/1(cfblk2) -> cfblk5/2
  cfblk7/1 -> cfblk12/1(cfblk1)
  cfblk12/2(cfblk12) -> cfblk6/1
  cfblk6/1 -> cfblk14/1(cfblk1)
  cfblk1/1 -> cfblk4/1
  cfblk5/1 -> cfblk2/1
  cfblk13/2(cfblk10) -> cfblk14/2(cfblk10)
  cfblk8/1 -> cfblk12/2(cfblk11)
  cfblk13/3(cfblk11) -> cfblk14/3(cfblk11), cfblk14/5(cfblk13)
  cfblk3/1 -> cfblk17/1
  cfblk17/1 -> cfblk13/2(cfblk8)

== system sampleModel106/cfblk81/cfblk8/cfblk4 ==
  cfblk1 : Inport
  cfblk6 : Inport  Port=2
  cfblk7 : Inport  Port=3
  cfblk{10..13} (4 alike) : Delay  SampleTime=1
  cfblk3 : simulink/Discrete/Transfer Fcn Lead or Lag  PoleZ=0.95  ZeroZ=0.75  ICPrevOutput=0.0  ICPrevInput=0.0  DoSatur=off
      settings: SourceProductBaseCode=SL
  cfblk4 : Subsystem
  cfblk5 : If  IfExpression=u1 >= 0  SampleTime=1
  cfblk8 : Subsystem  TreatAsAtomicUnit=on
  cfblk9 : Subsystem  TreatAsAtomicUnit=on
  cfblk2 : Outport
  wires:
  cfblk7/1 -> cfblk4/1(cfblk1)
  cfblk1/1 -> cfblk9/1(cfblk1), cfblk8/2(cfblk13)
  cfblk8/1(cfblk2) -> cfblk2/1
  cfblk6/1 -> cfblk4/2(cfblk12), cfblk8/1(cfblk1)
  cfblk3/1 -> cfblk10/1, cfblk11/1
  cfblk9/1(cfblk2) -> cfblk3/1
  cfblk8/3(cfblk16) -> cfblk4/3(cfblk13)
  cfblk5/1 -> cfblk8/Action
  cfblk5/2 -> cfblk9/Action
  cfblk10/1 -> cfblk9/3(cfblk9)
  cfblk11/1 -> cfblk8/3(cfblk14)
  cfblk8/2(cfblk15) -> cfblk12/1
  cfblk12/1 -> cfblk9/2(cfblk8)
  cfblk4/1(cfblk2) -> cfblk13/1
  cfblk13/1 -> cfblk5/1

== system sampleModel106/cfblk81/cfblk8/cfblk5 ==
  cfblk1 : Inport
  cfblk9 : Inport  Port=2
  cfblk{10..13} (4 alike) : Delay  SampleTime=1
  cfblk3 : simulink/Discrete/Tapped Delay  vinit=0.0  samptime=-1  NumDelays=1  DelayOrder=Oldest  includeCurrent=off
  cfblk4 : DiscreteIntegrator  ICPrevOutput=DiscIntNeverNeededParam  ICPrevScaledInput=DiscIntNeverNeededParam
  cfblk5 : DotProduct  OutDataTypeStr=Inherit: Inherit via internal rule
  cfblk6 : Constant  Value=[169771499.383824]  SampleTime=1
  cfblk7 : Subsystem
  cfblk8 : Subsystem
  cfblk2 : Outport
  wires:
  cfblk5/1 -> cfblk4/1
  cfblk6/1 -> cfblk5/1
  cfblk9/1 -> cfblk2/1
  cfblk8/1(cfblk2) -> cfblk3/1
  cfblk7/1(cfblk2) -> cfblk5/2
  cfblk4/1 -> cfblk8/2(cfblk9), cfblk8/4(cfblk11)
  cfblk7/2(cfblk14) -> cfblk8/3(cfblk10)
  cfblk1/1 -> cfblk7/1(cfblk1)
  cfblk3/1 -> cfblk10/1
  cfblk10/1 -> cfblk8/1(cfblk1)
  cfblk8/2(cfblk12) -> cfblk11/1
  cfblk11/1 -> cfblk7/2(cfblk11)
  cfblk8/3(cfblk13) -> cfblk12/1
  cfblk12/1 -> cfblk7/3(cfblk12)
  cfblk8/4(cfblk14) -> cfblk13/1
  cfblk13/1 -> cfblk7/4(cfblk13)

== system sampleModel106/cfblk81/cfblk8/cfblk6 ==
  cfblk1 : Inport
  cfblk12 : Inport  Port=2
  cfblk13 : Inport  Port=3
  cfblk14 : Inport  Port=4
  cfblk10 : Constant  Value=[156686469.491187]  SampleTime=1
  cfblk11 : Subsystem
  cfblk15 : Delay  SampleTime=1
  cfblk16 : Delay  SampleTime=1
  cfblk3 : DiscreteIntegrator  ICPrevOutput=DiscIntNeverNeededParam  ICPrevScaledInput=DiscIntNeverNeededParam
  cfblk4 : Polyval  Coefs=[ +2.081618890e-019, -1.441693666e-014, +4.719686976e-010, -8.536869453e-006, +1.621573104e-001, -8.087801117e+001 ]
  cfblk5 : Signum
  cfblk6 : simulink/Math Operations/MinMax Running Resettable  Function=min  vinit=0.0
  cfblk7 : Rounding
  cfblk8 : Sin  TimeSource=Use external signal  SampleTime=0
  cfblk9 : Sum  Inputs=+-
  cfblk2 : Outport
  wires:
  cfblk5/1 -> cfblk7/1
  cfblk12/1 -> cfblk5/1
  cfblk6/1 -> cfblk9/1
  cfblk9/1 -> cfblk11/1(cfblk1)
  cfblk13/1 -> cfblk4/1
  cfblk14/1 -> cfblk2/1
  cfblk11/1(cfblk2) -> cfblk8/1
  cfblk7/1 -> cfblk6/1
  cfblk10/1 -> cfblk6/2
  cfblk1/1 -> cfblk3/1
  cfblk8/1 -> cfblk15/1
  cfblk15/1 -> cfblk11/2(cfblk8)
  cfblk11/2(cfblk9) -> cfblk16/1
  cfblk16/1 -> cfblk9/2

== system sampleModel106/cfblk82/cfblk7/cfblk12 ==
  cfblk1 : Inport
  cfblk8 : Inport  Port=2
  Action Port : ActionPort  ActionPortLabel=if(u1 >= 0)
  cfblk10 : Delay
  cfblk3 : Delay  ShowEnablePort=on
      settings: InputPortMap=u0,e6
  cfblk4 : Product  Inputs=*
  cfblk5 : Reshape
  cfblk6 : Subsystem
  cfblk7 : Subsystem
  cfblk9 : Delay
  cfblk2 : Outport
  wires:
  cfblk4/1 -> cfblk7/1(cfblk1), cfblk6/3(cfblk14)
  cfblk1/1 -> cfblk5/1
  cfblk5/1 -> cfblk4/1
  cfblk7/1(cfblk2) -> cfblk6/1(cfblk1)
  cfblk8/1 -> cfblk6/2(cfblk13)
  cfblk7/2(cfblk16) -> cfblk3/1
  cfblk7/3(cfblk17) -> cfblk3/2
  cfblk6/2(cfblk15) -> cfblk2/1
  cfblk6/1(cfblk2) -> cfblk9/1
  cfblk9/1 -> cfblk7/2(cfblk14)
  cfblk3/1 -> cfblk10/1
  cfblk10/1 -> cfblk7/3(cfblk15)

== system sampleModel106/cfblk82/cfblk7/cfblk13 ==
  cfblk1 : Inport
  cfblk7 : Inport  Port=2
  cfblk8 : Inport  Port=3
  Action Port : ActionPort  ActionPortLabel=else
  cfblk3 : slpidlib/PID Controller  Controller=PID  Form=Parallel  TimeDomain=Discrete-time  UseExternalTs=off  SampleTime=-1  IntegratorMethod=Forward Euler  FilterMethod=Forward Euler  ControllerParametersSource=internal  P=1  I=1  UseKiTs=off  D=0  N=100  UseFilter=on  TunerSelectOption=Transfer Function Based (PID Tuner App)  InitialConditionSource=internal  InitialConditionForIntegrator=0  InitialConditionForFilter=0  DifferentiatorICPrevScaledInput=0  ExternalReset=none  TrackingMode=off  Kt=1  LimitOutput=off  SatLimitsSource=internal  UpperSaturationLimit=inf  LowerSaturationLimit=-inf  LinearizeAsGain=off  AntiWindupMode=none  Kb=1  POutMin=[]  POutMax=[]  IOutMin=[]  IOutMax=[]  DOutMin=[]  DOutMax=[]  NOutMin=[]  NOutMax=[]  SumOutMin=[]  SumOutMax=[]  SaturationOutMin=[]  SaturationOutMax=[]  PParamMin=[]  PParamMax=[]  IParamMin=[]  IParamMax=[]  DParamMin=[]  DParamMax=[]  NParamMin=[]  NParamMax=[]  KbParamMin=[]  KbParamMax=[]  KtParamMin=[]  KtParamMax=[]  KbOutMin=[]  KbOutMax=[]  KtOutMin=[]  KtOutMax=[]  IntegratorOutMin=[]  IntegratorOutMax=[]  FilterOutMin=[]  FilterOutMax=[]  SumI1OutMin=[]  SumI1OutMax=[]  SumI2OutMin=[]  SumI2OutMax=[]  SumI3OutMin=[]  SumI3OutMax=[]  SumI4OutMin=[]  SumI4OutMax=[]  SumDOutMin=[]  SumDOutMax=[]  DifferentiatorOutMin=[]  DifferentiatorOutMax=[]  FilterDiffOutCoefMin=[]  FilterDiffOutCoefMax=[]  ReciprocalOutMin=[]  ReciprocalOutMax=[]  SumDenOutMin=[]  SumDenOutMax=[]  SumNumOutMin=[]  SumNumOutMax=[]  DivideOutMin=[]  DivideOutMax=[]  UdiffTsProdOutMin=[]  UdiffTsProdOutMax=[]  NTsProdOutMin=[]  NTsProdOutMax=[]  UintegralTsProdOutMin=[]  UintegralTsProdOutMax=[]  UngainTsProdOutMin=[]  UngainTsProdOutMax=[]  IntegratorContinuousStateAttributes=''  IntegratorStateMustResolveToSignalObject=off  IntegratorRTWStateStorageClass=Auto  FilterContinuousStateAttributes=''  FilterStateMustResolveToSignalObject=off  FilterRTWStateStorageClass=Auto  ParallelPVariant=InternalParameters  IdealPVariant=Disabled  IVariant=InternalParameters  DVariant=InternalParameters  IntegratorVariant=Discrete  SatVariant=Disabled  AWVariant=Passthrough  PCopyVariant=Disabled  TRVariant=Disabled  FdbkBlocksVariant=Forward  IdealPFdbkVariant=Disabled  SatFdbkVariant=Disabled  DerivativeFilterVariant=ForwardEulerFilter  NVariant=InternalParameters  NCopyVariant=Disabled  FilterICVariant=InternalICsFilter  IntegratorICVariant=InternalICs  ExternalResetVariant=Disabled  TRSumVariant=Passthrough  SumFdbkVariant=Disabled  SumVariant=Sum_PID  TsampFilterVariant=InternalTs  TsampNgainVariant=Passthrough  TsampIntegralVariant=Passthrough  ExternalSaturationOutDataTypeStr=Inherit: Same as second input  aMode=0
  cfblk4 : Sum  Inputs=+-
  cfblk5 : Product
  cfblk6 : Subsystem
  cfblk2 : Outport
  cfblk9 : Outport  Port=2
  wires:
  cfblk5/1 -> cfblk3/1
  cfblk1/1 -> cfblk4/1, cfblk6/2(cfblk9)
  cfblk4/1 -> cfblk5/1
  cfblk3/1 -> cfblk2/1
  cfblk6/1(cfblk2) -> cfblk4/2
  cfblk8/1 -> cfblk6/1(cfblk1)
  cfblk7/1 -> cfblk5/2
  cfblk6/2(cfblk10) -> cfblk9/1

== system sampleModel106/cfblk82/cfblk7/cfblk6 ==
  cfblk1 : Inport
  cfblk12 : Inport  Port=2
  cfblk13 : Inport  Port=3
  cfblk10 : Subsystem
  cfblk11 : Subsystem
  cfblk14 : Delay  SampleTime=1
  cfblk15 : Delay  SampleTime=1
  cfblk16 : Delay  SampleTime=1
  cfblk3 : simulink/Math Operations/Slider Gain  gain=1  low=0  high=2
  cfblk4 : Polyval  Coefs=[ +2.081618890e-019, -1.441693666e-014, +4.719686976e-010, -8.536869453e-006, +1.621573104e-001, -8.087801117e+001 ]
  cfblk5 : Reshape
  cfblk6 : Sum  Inputs=+
  cfblk7 : Rounding
  cfblk8 : Subsystem
  cfblk9 : Subsystem
  cfblk2 : Outport
  wires:
  cfblk4/1 -> cfblk5/1
  cfblk7/1 -> cfblk11/1(cfblk1)
  cfblk10/1(cfblk2) -> cfblk8/1(cfblk1)
  cfblk12/1 -> cfblk6/1
  cfblk3/1 -> cfblk7/1
  cfblk5/1 -> cfblk9/1(cfblk1)
  cfblk6/1 -> cfblk10/2(cfblk13)
  cfblk8/1(cfblk2) -> cfblk3/1
  cfblk13/1 -> cfblk2/1
  cfblk1/1 -> cfblk10/4(cfblk15)
  cfblk11/1(cfblk2) -> cfblk14/1
  cfblk14/1 -> cfblk10/1(cfblk1)
  cfblk11/2(cfblk10) -> cfblk15/1
  cfblk15/1 -> cfblk10/3(cfblk14)
  cfblk9/1(cfblk2) -> cfblk16/1
  cfblk16/1 -> cfblk4/1
